simulink model "TEModel"  (Simulink 8.3)
settings: Solver=ode1  SolverMode=SingleTasking  StartTime=0.0  StopTime=72  FixedStep=Ts_base  MaxStep=Ts_base  MinStep=1e-6  RelTol=1e-6
PreLoadFcn:
  | initModel
StopFcn:
  | TEplot
undefined symbols (not defined in the file): Ts_base, Ts_save
libraries: VAlib x28, TElib x18
(part 8 of 9)

== system TEModel/TE Plant/xmeas atk block/xmeas11 attack controller/Attack Type Controller ==
  note: 1) Only subsystems can be added as variant choices at this level
      | 2) Blocks cannot be connected at this level as connectivity is
      | automatically determined at simulation, based on the active variant
  normal : Inport
  faked : Inport  Port=2
  interval forward controller : Subsystem  VariantControl=interval_forward_controller
      mask Display:
      | disp('IFC')
      | port_label('input', 1, 'normal in')
      | port_label('input', 2, 'faked in')
      | port_label('output', 1, 'out')
  normal forward controller : Subsystem  VariantControl=normal_forward_controller
      mask Display:
      | disp('NFC')
      | port_label('input', 1, 'normal in')
      | port_label('input', 2, 'faked in')
      | port_label('output', 1, 'out')
  periodical forward controller : Subsystem  VariantControl=periodical_forward_controller
      mask Display:
      | disp('PFC')
      | port_label('input', 1, 'normal in')
      | port_label('input', 2, 'faked in')
      | port_label('output', 1, 'out')
  step forward controller : Subsystem  VariantControl=step_forward_controller
      mask Display:
      | disp('SFC')
      | port_label('input', 1, 'normal in')
      | port_label('input', 2, 'faked in')
      | port_label('output', 1, 'out')
  output : Outport

== system TEModel/TE Plant/xmeas atk block/xmeas12 attack controller/Attack Type Controller ==
  note: 1) Only subsystems can be added as variant choices at this level
      | 2) Blocks cannot be connected at this level as connectivity is
      | automatically determined at simulation, based on the active variant
  normal : Inport
  faked : Inport  Port=2
  interval forward controller : Subsystem  VariantControl=interval_forward_controller
      mask Display:
      | disp('IFC')
      | port_label('input', 1, 'normal in')
      | port_label('input', 2, 'faked in')
      | port_label('output', 1, 'out')
  normal forward controller : Subsystem  VariantControl=normal_forward_controller
      mask Display:
      | disp('NFC')
      | port_label('input', 1, 'normal in')
      | port_label('input', 2, 'faked in')
      | port_label('output', 1, 'out')
  periodical forward controller : Subsystem  VariantControl=periodical_forward_controller
      mask Display:
      | disp('PFC')
      | port_label('input', 1, 'normal in')
      | port_label('input', 2, 'faked in')
      | port_label('output', 1, 'out')
  step forward controller : Subsystem  VariantControl=step_forward_controller
      mask Display:
      | disp('SFC')
      | port_label('input', 1, 'normal in')
      | port_label('input', 2, 'faked in')
      | port_label('output', 1, 'out')
  output : Outport

== system TEModel/TE Plant/xmeas atk block/xmeas14 attack controller/Attack Type Controller ==
  note: 1) Only subsystems can be added as variant choices at this level
      | 2) Blocks cannot be connected at this level as connectivity is
      | automatically determined at simulation, based on the active variant
  normal : Inport
  faked : Inport  Port=2
  interval forward controller : Subsystem  VariantControl=interval_forward_controller
      mask Display:
      | disp('IFC')
      | port_label('input', 1, 'normal in')
      | port_label('input', 2, 'faked in')
      | port_label('output', 1, 'out')
  normal forward controller : Subsystem  VariantControl=normal_forward_controller
      mask Display:
      | disp('NFC')
      | port_label('input', 1, 'normal in')
      | port_label('input', 2, 'faked in')
      | port_label('output', 1, 'out')
  periodical forward controller : Subsystem  VariantControl=periodical_forward_controller
      mask Display:
      | disp('PFC')
      | port_label('input', 1, 'normal in')
      | port_label('input', 2, 'faked in')
      | port_label('output', 1, 'out')
  step forward controller : Subsystem  VariantControl=step_forward_controller
      mask Display:
      | disp('SFC')
      | port_label('input', 1, 'normal in')
      | port_label('input', 2, 'faked in')
      | port_label('output', 1, 'out')
  output : Outport

== system TEModel/TE Plant/xmeas atk block/xmeas15 attack controller/Attack Type Controller ==
  note: 1) Only subsystems can be added as variant choices at this level
      | 2) Blocks cannot be connected at this level as connectivity is
      | automatically determined at simulation, based on the active variant
  normal : Inport
  faked : Inport  Port=2
  interval forward controller : Subsystem  VariantControl=interval_forward_controller
      mask Display:
      | disp('IFC')
      | port_label('input', 1, 'normal in')
      | port_label('input', 2, 'faked in')
      | port_label('output', 1, 'out')
  normal forward controller : Subsystem  VariantControl=normal_forward_controller
      mask Display:
      | disp('NFC')
      | port_label('input', 1, 'normal in')
      | port_label('input', 2, 'faked in')
      | port_label('output', 1, 'out')
  periodical forward controller : Subsystem  VariantControl=periodical_forward_controller
      mask Display:
      | disp('PFC')
      | port_label('input', 1, 'normal in')
      | port_label('input', 2, 'faked in')
      | port_label('output', 1, 'out')
  step forward controller : Subsystem  VariantControl=step_forward_controller
      mask Display:
      | disp('SFC')
      | port_label('input', 1, 'normal in')
      | port_label('input', 2, 'faked in')
      | port_label('output', 1, 'out')
  output : Outport

== system TEModel/TE Plant/xmeas atk block/xmeas17 attack controller/Attack Type Controller ==
  note: 1) Only subsystems can be added as variant choices at this level
      | 2) Blocks cannot be connected at this level as connectivity is
      | automatically determined at simulation, based on the active variant
  normal : Inport
  faked : Inport  Port=2
  interval forward controller : Subsystem  VariantControl=interval_forward_controller
      mask Display:
      | disp('IFC')
      | port_label('input', 1, 'normal in')
      | port_label('input', 2, 'faked in')
      | port_label('output', 1, 'out')
  normal forward controller : Subsystem  VariantControl=normal_forward_controller
      mask Display:
      | disp('NFC')
      | port_label('input', 1, 'normal in')
      | port_label('input', 2, 'faked in')
      | port_label('output', 1, 'out')
  periodical forward controller : Subsystem  VariantControl=periodical_forward_controller
      mask Display:
      | disp('PFC')
      | port_label('input', 1, 'normal in')
      | port_label('input', 2, 'faked in')
      | port_label('output', 1, 'out')
  step forward controller : Subsystem  VariantControl=step_forward_controller
      mask Display:
      | disp('SFC')
      | port_label('input', 1, 'normal in')
      | port_label('input', 2, 'faked in')
      | port_label('output', 1, 'out')
  output : Outport

== system TEModel/TE Plant/xmeas atk block/xmeas2 attack controller/Attack Type Controller ==
  note: 1) Only subsystems can be added as variant choices at this level
      | 2) Blocks cannot be connected at this level as connectivity is
      | automatically determined at simulation, based on the active variant
  normal : Inport
  faked : Inport  Port=2
  interval forward controller : Subsystem  VariantControl=interval_forward_controller
      mask Display:
      | disp('IFC')
      | port_label('input', 1, 'normal in')
      | port_label('input', 2, 'faked in')
      | port_label('output', 1, 'out')
  normal forward controller : Subsystem  VariantControl=normal_forward_controller
      mask Display:
      | disp('NFC')
      | port_label('input', 1, 'normal in')
      | port_label('input', 2, 'faked in')
      | port_label('output', 1, 'out')
  periodical forward controller : Subsystem  VariantControl=periodical_forward_controller
      mask Display:
      | disp('PFC')
      | port_label('input', 1, 'normal in')
      | port_label('input', 2, 'faked in')
      | port_label('output', 1, 'out')
  step forward controller : Subsystem  VariantControl=step_forward_controller
      mask Display:
      | disp('SFC')
      | port_label('input', 1, 'normal in')
      | port_label('input', 2, 'faked in')
      | port_label('output', 1, 'out')
  output : Outport

== system TEModel/TE Plant/xmeas atk block/xmeas3 attack controller/Attack Type Controller ==
  note: 1) Only subsystems can be added as variant choices at this level
      | 2) Blocks cannot be connected at this level as connectivity is
      | automatically determined at simulation, based on the active variant
  normal : Inport
  faked : Inport  Port=2
  interval forward controller : Subsystem  VariantControl=interval_forward_controller
      mask Display:
      | disp('IFC')
      | port_label('input', 1, 'normal in')
      | port_label('input', 2, 'faked in')
      | port_label('output', 1, 'out')
  normal forward controller : Subsystem  VariantControl=normal_forward_controller
      mask Display:
      | disp('NFC')
      | port_label('input', 1, 'normal in')
      | port_label('input', 2, 'faked in')
      | port_label('output', 1, 'out')
  periodical forward controller : Subsystem  VariantControl=periodical_forward_controller
      mask Display:
      | disp('PFC')
      | port_label('input', 1, 'normal in')
      | port_label('input', 2, 'faked in')
      | port_label('output', 1, 'out')
  step forward controller : Subsystem  VariantControl=step_forward_controller
      mask Display:
      | disp('SFC')
      | port_label('input', 1, 'normal in')
      | port_label('input', 2, 'faked in')
      | port_label('output', 1, 'out')
  output : Outport

== system TEModel/TE Plant/xmeas atk block/xmeas31 attack controller/Attack Type Controller ==
  note: 1) Only subsystems can be added as variant choices at this level
      | 2) Blocks cannot be connected at this level as connectivity is
      | automatically determined at simulation, based on the active variant
  normal : Inport
  faked : Inport  Port=2
  interval forward controller : Subsystem  VariantControl=interval_forward_controller
      mask Display:
      | disp('IFC')
      | port_label('input', 1, 'normal in')
      | port_label('input', 2, 'faked in')
      | port_label('output', 1, 'out')
  normal forward controller : Subsystem  VariantControl=normal_forward_controller
      mask Display:
      | disp('NFC')
      | port_label('input', 1, 'normal in')
      | port_label('input', 2, 'faked in')
      | port_label('output', 1, 'out')
  periodical forward controller : Subsystem  VariantControl=periodical_forward_controller
      mask Display:
      | disp('PFC')
      | port_label('input', 1, 'normal in')
      | port_label('input', 2, 'faked in')
      | port_label('output', 1, 'out')
  step forward controller : Subsystem  VariantControl=step_forward_controller
      mask Display:
      | disp('SFC')
      | port_label('input', 1, 'normal in')
      | port_label('input', 2, 'faked in')
      | port_label('output', 1, 'out')
  output : Outport

== system TEModel/TE Plant/xmeas atk block/xmeas4 attack controller/Attack Type Controller ==
  note: 1) Only subsystems can be added as variant choices at this level
      | 2) Blocks cannot be connected at this level as connectivity is
      | automatically determined at simulation, based on the active variant
  normal : Inport
  faked : Inport  Port=2
  interval forward controller : Subsystem  VariantControl=interval_forward_controller
      mask Display:
      | disp('IFC')
      | port_label('input', 1, 'normal in')
      | port_label('input', 2, 'faked in')
      | port_label('output', 1, 'out')
  normal forward controller : Subsystem  VariantControl=normal_forward_controller
      mask Display:
      | disp('NFC')
      | port_label('input', 1, 'normal in')
      | port_label('input', 2, 'faked in')
      | port_label('output', 1, 'out')
  periodical forward controller : Subsystem  VariantControl=periodical_forward_controller
      mask Display:
      | disp('PFC')
      | port_label('input', 1, 'normal in')
      | port_label('input', 2, 'faked in')
      | port_label('output', 1, 'out')
  step forward controller : Subsystem  VariantControl=step_forward_controller
      mask Display:
      | disp('SFC')
      | port_label('input', 1, 'normal in')
      | port_label('input', 2, 'faked in')
      | port_label('output', 1, 'out')
  output : Outport

== system TEModel/TE Plant/xmeas atk block/xmeas40 attack controller/Attack Type Controller ==
  note: 1) Only subsystems can be added as variant choices at this level
      | 2) Blocks cannot be connected at this level as connectivity is
      | automatically determined at simulation, based on the active variant
  normal : Inport
  faked : Inport  Port=2
  interval forward controller : Subsystem  VariantControl=interval_forward_controller
      mask Display:
      | disp('IFC')
      | port_label('input', 1, 'normal in')
      | port_label('input', 2, 'faked in')
      | port_label('output', 1, 'out')
  normal forward controller : Subsystem  VariantControl=normal_forward_controller
      mask Display:
      | disp('NFC')
      | port_label('input', 1, 'normal in')
      | port_label('input', 2, 'faked in')
      | port_label('output', 1, 'out')
  periodical forward controller : Subsystem  VariantControl=periodical_forward_controller
      mask Display:
      | disp('PFC')
      | port_label('input', 1, 'normal in')
      | port_label('input', 2, 'faked in')
      | port_label('output', 1, 'out')
  step forward controller : Subsystem  VariantControl=step_forward_controller
      mask Display:
      | disp('SFC')
      | port_label('input', 1, 'normal in')
      | port_label('input', 2, 'faked in')
      | port_label('output', 1, 'out')
  output : Outport

== system TEModel/TE Plant/xmeas atk block/xmeas5 attack controller/Attack Type Controller ==
  note: 1) Only subsystems can be added as variant choices at this level
      | 2) Blocks cannot be connected at this level as connectivity is
      | automatically determined at simulation, based on the active variant
  normal : Inport
  faked : Inport  Port=2
  interval forward controller : Subsystem  VariantControl=interval_forward_controller
      mask Display:
      | disp('IFC')
      | port_label('input', 1, 'normal in')
      | port_label('input', 2, 'faked in')
      | port_label('output', 1, 'out')
  normal forward controller : Subsystem  VariantControl=normal_forward_controller
      mask Display:
      | disp('NFC')
      | port_label('input', 1, 'normal in')
      | port_label('input', 2, 'faked in')
      | port_label('output', 1, 'out')
  periodical forward controller : Subsystem  VariantControl=periodical_forward_controller
      mask Display:
      | disp('PFC')
      | port_label('input', 1, 'normal in')
      | port_label('input', 2, 'faked in')
      | port_label('output', 1, 'out')
  step forward controller : Subsystem  VariantControl=step_forward_controller
      mask Display:
      | disp('SFC')
      | port_label('input', 1, 'normal in')
      | port_label('input', 2, 'faked in')
      | port_label('output', 1, 'out')
  output : Outport

== system TEModel/TE Plant/xmeas atk block/xmeas7 attack controller/Attack Type Controller ==
  note: 1) Only subsystems can be added as variant choices at this level
      | 2) Blocks cannot be connected at this level as connectivity is
      | automatically determined at simulation, based on the active variant
  normal : Inport
  faked : Inport  Port=2
  interval forward controller : Subsystem  VariantControl=interval_forward_controller
      mask Display:
      | disp('IFC')
      | port_label('input', 1, 'normal in')
      | port_label('input', 2, 'faked in')
      | port_label('output', 1, 'out')
  normal forward controller : Subsystem  VariantControl=normal_forward_controller
      mask Display:
      | disp('NFC')
      | port_label('input', 1, 'normal in')
      | port_label('input', 2, 'faked in')
      | port_label('output', 1, 'out')
  periodical forward controller : Subsystem  VariantControl=periodical_forward_controller
      mask Display:
      | disp('PFC')
      | port_label('input', 1, 'normal in')
      | port_label('input', 2, 'faked in')
      | port_label('output', 1, 'out')
  step forward controller : Subsystem  VariantControl=step_forward_controller
      mask Display:
      | disp('SFC')
      | port_label('input', 1, 'normal in')
      | port_label('input', 2, 'faked in')
      | port_label('output', 1, 'out')
  output : Outport

== system TEModel/TE Plant/xmeas atk block/xmeas8 attack controller/Attack Type Controller ==
  note: 1) Only subsystems can be added as variant choices at this level
      | 2) Blocks cannot be connected at this level as connectivity is
      | automatically determined at simulation, based on the active variant
  normal : Inport
  faked : Inport  Port=2
  interval forward controller : Subsystem  VariantControl=interval_forward_controller
      mask Display:
      | disp('IFC')
      | port_label('input', 1, 'normal in')
      | port_label('input', 2, 'faked in')
      | port_label('output', 1, 'out')
  normal forward controller : Subsystem  VariantControl=normal_forward_controller
      mask Display:
      | disp('NFC')
      | port_label('input', 1, 'normal in')
      | port_label('input', 2, 'faked in')
      | port_label('output', 1, 'out')
  periodical forward controller : Subsystem  VariantControl=periodical_forward_controller
      mask Display:
      | disp('PFC')
      | port_label('input', 1, 'normal in')
      | port_label('input', 2, 'faked in')
      | port_label('output', 1, 'out')
  step forward controller : Subsystem  VariantControl=step_forward_controller
      mask Display:
      | disp('SFC')
      | port_label('input', 1, 'normal in')
      | port_label('input', 2, 'faked in')
      | port_label('output', 1, 'out')
  output : Outport

== system TEModel/TE Plant/xmeas atk block/xmeas9 attack controller/Attack Type Controller ==
  note: 1) Only subsystems can be added as variant choices at this level
      | 2) Blocks cannot be connected at this level as connectivity is
      | automatically determined at simulation, based on the active variant
  normal : Inport
  faked : Inport  Port=2
  interval forward controller : Subsystem  VariantControl=interval_forward_controller
      mask Display:
      | disp('IFC')
      | port_label('input', 1, 'normal in')
      | port_label('input', 2, 'faked in')
      | port_label('output', 1, 'out')
  normal forward controller : Subsystem  VariantControl=normal_forward_controller
      mask Display:
      | disp('NFC')
      | port_label('input', 1, 'normal in')
      | port_label('input', 2, 'faked in')
      | port_label('output', 1, 'out')
  periodical forward controller : Subsystem  VariantControl=periodical_forward_controller
      mask Display:
      | disp('PFC')
      | port_label('input', 1, 'normal in')
      | port_label('input', 2, 'faked in')
      | port_label('output', 1, 'out')
  step forward controller : Subsystem  VariantControl=step_forward_controller
      mask Display:
      | disp('SFC')
      | port_label('input', 1, 'normal in')
      | port_label('input', 2, 'faked in')
      | port_label('output', 1, 'out')
  output : Outport

== system TEModel/TE Plant/xmv atk block/xmv1 attack controller/Attack Type Controller ==
  note: 1) Only subsystems can be added as variant choices at this level
      | 2) Blocks cannot be connected at this level as connectivity is
      | automatically determined at simulation, based on the active variant
  normal : Inport
  faked : Inport  Port=2
  interval forward controller : Subsystem  VariantControl=interval_forward_controller
      mask Display:
      | disp('IFC')
      | port_label('input', 1, 'normal in')
      | port_label('input', 2, 'faked in')
      | port_label('output', 1, 'out')
  normal forward controller : Subsystem  VariantControl=normal_forward_controller
      mask Display:
      | disp('NFC')
      | port_label('input', 1, 'normal in')
      | port_label('input', 2, 'faked in')
      | port_label('output', 1, 'out')
  periodical forward controller : Subsystem  VariantControl=periodical_forward_controller
      mask Display:
      | disp('PFC')
      | port_label('input', 1, 'normal in')
      | port_label('input', 2, 'faked in')
      | port_label('output', 1, 'out')
  step forward controller : Subsystem  VariantControl=step_forward_controller
      mask Display:
      | disp('SFC')
      | port_label('input', 1, 'normal in')
      | port_label('input', 2, 'faked in')
      | port_label('output', 1, 'out')
  output : Outport

== system TEModel/TE Plant/xmv atk block/xmv10 attack controller/Attack Type Controller ==
  note: 1) Only subsystems can be added as variant choices at this level
      | 2) Blocks cannot be connected at this level as connectivity is
      | automatically determined at simulation, based on the active variant
  normal : Inport
  faked : Inport  Port=2
  interval forward controller : Subsystem  VariantControl=interval_forward_controller
      mask Display:
      | disp('IFC')
      | port_label('input', 1, 'normal in')
      | port_label('input', 2, 'faked in')
      | port_label('output', 1, 'out')
  normal forward controller : Subsystem  VariantControl=normal_forward_controller
      mask Display:
      | disp('NFC')
      | port_label('input', 1, 'normal in')
      | port_label('input', 2, 'faked in')
      | port_label('output', 1, 'out')
  periodical forward controller : Subsystem  VariantControl=periodical_forward_controller
      mask Display:
      | disp('PFC')
      | port_label('input', 1, 'normal in')
      | port_label('input', 2, 'faked in')
      | port_label('output', 1, 'out')
  step forward controller : Subsystem  VariantControl=step_forward_controller
      mask Display:
      | disp('SFC')
      | port_label('input', 1, 'normal in')
      | port_label('input', 2, 'faked in')
      | port_label('output', 1, 'out')
  output : Outport

== system TEModel/TE Plant/xmv atk block/xmv11 attack controller/Attack Type Controller ==
  note: 1) Only subsystems can be added as variant choices at this level
      | 2) Blocks cannot be connected at this level as connectivity is
      | automatically determined at simulation, based on the active variant
  normal : Inport
  faked : Inport  Port=2
  interval forward controller : Subsystem  VariantControl=interval_forward_controller
      mask Display:
      | disp('IFC')
      | port_label('input', 1, 'normal in')
      | port_label('input', 2, 'faked in')
      | port_label('output', 1, 'out')
  normal forward controller : Subsystem  VariantControl=normal_forward_controller
      mask Display:
      | disp('NFC')
      | port_label('input', 1, 'normal in')
      | port_label('input', 2, 'faked in')
      | port_label('output', 1, 'out')
  periodical forward controller : Subsystem  VariantControl=periodical_forward_controller
      mask Display:
      | disp('PFC')
      | port_label('input', 1, 'normal in')
      | port_label('input', 2, 'faked in')
      | port_label('output', 1, 'out')
  step forward controller : Subsystem  VariantControl=step_forward_controller
      mask Display:
      | disp('SFC')
      | port_label('input', 1, 'normal in')
      | port_label('input', 2, 'faked in')
      | port_label('output', 1, 'out')
  output : Outport

== system TEModel/TE Plant/xmv atk block/xmv12 attack controller/Attack Type Controller ==
  note: 1) Only subsystems can be added as variant choices at this level
      | 2) Blocks cannot be connected at this level as connectivity is
      | automatically determined at simulation, based on the active variant
  normal : Inport
  faked : Inport  Port=2
  interval forward controller : Subsystem  VariantControl=interval_forward_controller
      mask Display:
      | disp('IFC')
      | port_label('input', 1, 'normal in')
      | port_label('input', 2, 'faked in')
      | port_label('output', 1, 'out')
  normal forward controller : Subsystem  VariantControl=normal_forward_controller
      mask Display:
      | disp('NFC')
      | port_label('input', 1, 'normal in')
      | port_label('input', 2, 'faked in')
      | port_label('output', 1, 'out')
  periodical forward controller : Subsystem  VariantControl=periodical_forward_controller
      mask Display:
      | disp('PFC')
      | port_label('input', 1, 'normal in')
      | port_label('input', 2, 'faked in')
      | port_label('output', 1, 'out')
  step forward controller : Subsystem  VariantControl=step_forward_controller
      mask Display:
      | disp('SFC')
      | port_label('input', 1, 'normal in')
      | port_label('input', 2, 'faked in')
      | port_label('output', 1, 'out')
  output : Outport

== system TEModel/TE Plant/xmv atk block/xmv2 attack controller/Attack Type Controller ==
  note: 1) Only subsystems can be added as variant choices at this level
      | 2) Blocks cannot be connected at this level as connectivity is
      | automatically determined at simulation, based on the active variant
  normal : Inport
  faked : Inport  Port=2
  interval forward controller : Subsystem  VariantControl=interval_forward_controller
      mask Display:
      | disp('IFC')
      | port_label('input', 1, 'normal in')
      | port_label('input', 2, 'faked in')
      | port_label('output', 1, 'out')
  normal forward controller : Subsystem  VariantControl=normal_forward_controller
      mask Display:
      | disp('NFC')
      | port_label('input', 1, 'normal in')
      | port_label('input', 2, 'faked in')
      | port_label('output', 1, 'out')
  periodical forward controller : Subsystem  VariantControl=periodical_forward_controller
      mask Display:
      | disp('PFC')
      | port_label('input', 1, 'normal in')
      | port_label('input', 2, 'faked in')
      | port_label('output', 1, 'out')
  step forward controller : Subsystem  VariantControl=step_forward_controller
      mask Display:
      | disp('SFC')
      | port_label('input', 1, 'normal in')
      | port_label('input', 2, 'faked in')
      | port_label('output', 1, 'out')
  output : Outport

== system TEModel/TE Plant/xmv atk block/xmv3 attack controller/Attack Type Controller ==
  note: 1) Only subsystems can be added as variant choices at this level
      | 2) Blocks cannot be connected at this level as connectivity is
      | automatically determined at simulation, based on the active variant
  normal : Inport
  faked : Inport  Port=2
  interval forward controller : Subsystem  VariantControl=interval_forward_controller
      mask Display:
      | disp('IFC')
      | port_label('input', 1, 'normal in')
      | port_label('input', 2, 'faked in')
      | port_label('output', 1, 'out')
  normal forward controller : Subsystem  VariantControl=normal_forward_controller
      mask Display:
      | disp('NFC')
      | port_label('input', 1, 'normal in')
      | port_label('input', 2, 'faked in')
      | port_label('output', 1, 'out')
  periodical forward controller : Subsystem  VariantControl=periodical_forward_controller
      mask Display:
      | disp('PFC')
      | port_label('input', 1, 'normal in')
      | port_label('input', 2, 'faked in')
      | port_label('output', 1, 'out')
  step forward controller : Subsystem  VariantControl=step_forward_controller
      mask Display:
      | disp('SFC')
      | port_label('input', 1, 'normal in')
      | port_label('input', 2, 'faked in')
      | port_label('output', 1, 'out')
  output : Outport

== system TEModel/TE Plant/xmv atk block/xmv4 attack controller/Attack Type Controller ==
  note: 1) Only subsystems can be added as variant choices at this level
      | 2) Blocks cannot be connected at this level as connectivity is
      | automatically determined at simulation, based on the active variant
  normal : Inport
  faked : Inport  Port=2
  interval forward controller : Subsystem  VariantControl=interval_forward_controller
      mask Display:
      | disp('IFC')
      | port_label('input', 1, 'normal in')
      | port_label('input', 2, 'faked in')
      | port_label('output', 1, 'out')
  normal forward controller : Subsystem  VariantControl=normal_forward_controller
      mask Display:
      | disp('NFC')
      | port_label('input', 1, 'normal in')
      | port_label('input', 2, 'faked in')
      | port_label('output', 1, 'out')
  periodical forward controller : Subsystem  VariantControl=periodical_forward_controller
      mask Display:
      | disp('PFC')
      | port_label('input', 1, 'normal in')
      | port_label('input', 2, 'faked in')
      | port_label('output', 1, 'out')
  step forward controller : Subsystem  VariantControl=step_forward_controller
      mask Display:
      | disp('SFC')
      | port_label('input', 1, 'normal in')
      | port_label('input', 2, 'faked in')
      | port_label('output', 1, 'out')
  output : Outport

== system TEModel/TE Plant/xmv atk block/xmv5 attack controller/Attack Type Controller ==
  note: 1) Only subsystems can be added as variant choices at this level
      | 2) Blocks cannot be connected at this level as connectivity is
      | automatically determined at simulation, based on the active variant
  normal : Inport
  faked : Inport  Port=2
  interval forward controller : Subsystem  VariantControl=interval_forward_controller
      mask Display:
      | disp('IFC')
      | port_label('input', 1, 'normal in')
      | port_label('input', 2, 'faked in')
      | port_label('output', 1, 'out')
  normal forward controller : Subsystem  VariantControl=normal_forward_controller
      mask Display:
      | disp('NFC')
      | port_label('input', 1, 'normal in')
      | port_label('input', 2, 'faked in')
      | port_label('output', 1, 'out')
  periodical forward controller : Subsystem  VariantControl=periodical_forward_controller
      mask Display:
      | disp('PFC')
      | port_label('input', 1, 'normal in')
      | port_label('input', 2, 'faked in')
      | port_label('output', 1, 'out')
  step forward controller : Subsystem  VariantControl=step_forward_controller
      mask Display:
      | disp('SFC')
      | port_label('input', 1, 'normal in')
      | port_label('input', 2, 'faked in')
      | port_label('output', 1, 'out')
  output : Outport

== system TEModel/TE Plant/xmv atk block/xmv6 attack controller/Attack Type Controller ==
  note: 1) Only subsystems can be added as variant choices at this level
      | 2) Blocks cannot be connected at this level as connectivity is
      | automatically determined at simulation, based on the active variant
  normal : Inport
  faked : Inport  Port=2
  interval forward controller : Subsystem  VariantControl=interval_forward_controller
      mask Display:
      | disp('IFC')
      | port_label('input', 1, 'normal in')
      | port_label('input', 2, 'faked in')
      | port_label('output', 1, 'out')
  normal forward controller : Subsystem  VariantControl=normal_forward_controller
      mask Display:
      | disp('NFC')
      | port_label('input', 1, 'normal in')
      | port_label('input', 2, 'faked in')
      | port_label('output', 1, 'out')
  periodical forward controller : Subsystem  VariantControl=periodical_forward_controller
      mask Display:
      | disp('PFC')
      | port_label('input', 1, 'normal in')
      | port_label('input', 2, 'faked in')
      | port_label('output', 1, 'out')
  step forward controller : Subsystem  VariantControl=step_forward_controller
      mask Display:
      | disp('SFC')
      | port_label('input', 1, 'normal in')
      | port_label('input', 2, 'faked in')
      | port_label('output', 1, 'out')
  output : Outport

== system TEModel/TE Plant/xmv atk block/xmv7 attack controller/Attack Type Controller ==
  note: 1) Only subsystems can be added as variant choices at this level
      | 2) Blocks cannot be connected at this level as connectivity is
      | automatically determined at simulation, based on the active variant
  normal : Inport
  faked : Inport  Port=2
  interval forward controller : Subsystem  VariantControl=interval_forward_controller
      mask Display:
      | disp('IFC')
      | port_label('input', 1, 'normal in')
      | port_label('input', 2, 'faked in')
      | port_label('output', 1, 'out')
  normal forward controller : Subsystem  VariantControl=normal_forward_controller
      mask Display:
      | disp('NFC')
      | port_label('input', 1, 'normal in')
      | port_label('input', 2, 'faked in')
      | port_label('output', 1, 'out')
  periodical forward controller : Subsystem  VariantControl=periodical_forward_controller
      mask Display:
      | disp('PFC')
      | port_label('input', 1, 'normal in')
      | port_label('input', 2, 'faked in')
      | port_label('output', 1, 'out')
  step forward controller : Subsystem  VariantControl=step_forward_controller
      mask Display:
      | disp('SFC')
      | port_label('input', 1, 'normal in')
      | port_label('input', 2, 'faked in')
      | port_label('output', 1, 'out')
  output : Outport

== system TEModel/TE Plant/xmv atk block/xmv8 attack controller/Attack Type Controller ==
  note: 1) Only subsystems can be added as variant choices at this level
      | 2) Blocks cannot be connected at this level as connectivity is
      | automatically determined at simulation, based on the active variant
  normal : Inport
  faked : Inport  Port=2
  interval forward controller : Subsystem  VariantControl=interval_forward_controller
      mask Display:
      | disp('IFC')
      | port_label('input', 1, 'normal in')
      | port_label('input', 2, 'faked in')
      | port_label('output', 1, 'out')
  normal forward controller : Subsystem  VariantControl=normal_forward_controller
      mask Display:
      | disp('NFC')
      | port_label('input', 1, 'normal in')
      | port_label('input', 2, 'faked in')
      | port_label('output', 1, 'out')
  periodical forward controller : Subsystem  VariantControl=periodical_forward_controller
      mask Display:
      | disp('PFC')
      | port_label('input', 1, 'normal in')
      | port_label('input', 2, 'faked in')
      | port_label('output', 1, 'out')
  step forward controller : Subsystem  VariantControl=step_forward_controller
      mask Display:
      | disp('SFC')
      | port_label('input', 1, 'normal in')
      | port_label('input', 2, 'faked in')
      | port_label('output', 1, 'out')
  output : Outport

== system TEModel/TE Plant/xmv atk block/xmv9 attack controller/Attack Type Controller ==
  note: 1) Only subsystems can be added as variant choices at this level
      | 2) Blocks cannot be connected at this level as connectivity is
      | automatically determined at simulation, based on the active variant
  normal : Inport
  faked : Inport  Port=2
  interval forward controller : Subsystem  VariantControl=interval_forward_controller
      mask Display:
      | disp('IFC')
      | port_label('input', 1, 'normal in')
      | port_label('input', 2, 'faked in')
      | port_label('output', 1, 'out')
  normal forward controller : Subsystem  VariantControl=normal_forward_controller
      mask Display:
      | disp('NFC')
      | port_label('input', 1, 'normal in')
      | port_label('input', 2, 'faked in')
      | port_label('output', 1, 'out')
  periodical forward controller : Subsystem  VariantControl=periodical_forward_controller
      mask Display:
      | disp('PFC')
      | port_label('input', 1, 'normal in')
      | port_label('input', 2, 'faked in')
      | port_label('output', 1, 'out')
  step forward controller : Subsystem  VariantControl=step_forward_controller
      mask Display:
      | disp('SFC')
      | port_label('input', 1, 'normal in')
      | port_label('input', 2, 'faked in')
      | port_label('output', 1, 'out')
  output : Outport

== system TEModel/TE Plant/xmeas atk block/xmeas1 attack controller/Attack Type Controller/interval forward controller ==
  normal : Inport
  faked : Inport  Port=2
  Impuls : VAlib/Impuls  amplitude=1  duration=duration  delay=start
  Switch : Switch  Criteria=u2 > Threshold
  output : Outport
  wires:
  faked/1 -> Switch/1
  normal/1 -> Switch/3
  Impuls/1 -> Switch/2
  Switch/1 -> output/1

== system TEModel/TE Plant/xmeas atk block/xmeas1 attack controller/Attack Type Controller/normal forward controller ==
  normal : Inport
  faked : Inport  Port=2
  Terminator : Terminator
  output : Outport
  wires:
  normal/1 -> output/1
  faked/1 -> Terminator/1

== system TEModel/TE Plant/xmeas atk block/xmeas1 attack controller/Attack Type Controller/periodical forward controller ==
  normal : Inport
  faked : Inport  Port=2
  Pulse Generator : DiscretePulseGenerator  PulseType=Time based  Period=duration + start  PulseWidth=100*duration/(duration + start)  PhaseDelay=start
  Switch : Switch  Criteria=u2 > Threshold
  output : Outport
  wires:
  faked/1 -> Switch/1
  normal/1 -> Switch/3
  Pulse Generator/1 -> Switch/2
  Switch/1 -> output/1

== system TEModel/TE Plant/xmeas atk block/xmeas1 attack controller/Attack Type Controller/step forward controller ==
  normal : Inport
  faked : Inport  Port=2
  Step : Step  Time=start  SampleTime=0
  Switch : Switch  Criteria=u2 > Threshold
  output : Outport
  wires:
  faked/1 -> Switch/1
  normal/1 -> Switch/3
  Step/1 -> Switch/2
  Switch/1 -> output/1

== system TEModel/TE Plant/xmeas atk block/xmeas10 attack controller/Attack Type Controller/interval forward controller ==
  normal : Inport
  faked : Inport  Port=2
  Impuls : VAlib/Impuls  amplitude=1  duration=duration  delay=start
  Switch : Switch  Criteria=u2 > Threshold
  output : Outport
  wires:
  faked/1 -> Switch/1
  normal/1 -> Switch/3
  Impuls/1 -> Switch/2
  Switch/1 -> output/1

== system TEModel/TE Plant/xmeas atk block/xmeas10 attack controller/Attack Type Controller/normal forward controller ==
  normal : Inport
  faked : Inport  Port=2
  Terminator : Terminator
  output : Outport
  wires:
  normal/1 -> output/1
  faked/1 -> Terminator/1

== system TEModel/TE Plant/xmeas atk block/xmeas10 attack controller/Attack Type Controller/periodical forward controller ==
  normal : Inport
  faked : Inport  Port=2
  Pulse Generator : DiscretePulseGenerator  PulseType=Time based  Period=duration + start  PulseWidth=100*duration/(duration + start)  PhaseDelay=start
  Switch : Switch  Criteria=u2 > Threshold
  output : Outport
  wires:
  faked/1 -> Switch/1
  normal/1 -> Switch/3
  Pulse Generator/1 -> Switch/2
  Switch/1 -> output/1

== system TEModel/TE Plant/xmeas atk block/xmeas10 attack controller/Attack Type Controller/step forward controller ==
  normal : Inport
  faked : Inport  Port=2
  Step : Step  Time=start  SampleTime=0
  Switch : Switch  Criteria=u2 > Threshold
  output : Outport
  wires:
  faked/1 -> Switch/1
  normal/1 -> Switch/3
  Step/1 -> Switch/2
  Switch/1 -> output/1

== system TEModel/TE Plant/xmeas atk block/xmeas11 attack controller/Attack Type Controller/interval forward controller ==
  normal : Inport
  faked : Inport  Port=2
  Impuls : VAlib/Impuls  amplitude=1  duration=duration  delay=start
  Switch : Switch  Criteria=u2 > Threshold
  output : Outport
  wires:
  faked/1 -> Switch/1
  normal/1 -> Switch/3
  Impuls/1 -> Switch/2
  Switch/1 -> output/1

== system TEModel/TE Plant/xmeas atk block/xmeas11 attack controller/Attack Type Controller/normal forward controller ==
  normal : Inport
  faked : Inport  Port=2
  Terminator : Terminator
  output : Outport
  wires:
  normal/1 -> output/1
  faked/1 -> Terminator/1

== system TEModel/TE Plant/xmeas atk block/xmeas11 attack controller/Attack Type Controller/periodical forward controller ==
  normal : Inport
  faked : Inport  Port=2
  Pulse Generator : DiscretePulseGenerator  PulseType=Time based  Period=duration + start  PulseWidth=100*duration/(duration + start)  PhaseDelay=start
  Switch : Switch  Criteria=u2 > Threshold
  output : Outport
  wires:
  faked/1 -> Switch/1
  normal/1 -> Switch/3
  Pulse Generator/1 -> Switch/2
  Switch/1 -> output/1

== system TEModel/TE Plant/xmeas atk block/xmeas11 attack controller/Attack Type Controller/step forward controller ==
  normal : Inport
  faked : Inport  Port=2
  Step : Step  Time=start  SampleTime=0
  Switch : Switch  Criteria=u2 > Threshold
  output : Outport
  wires:
  faked/1 -> Switch/1
  normal/1 -> Switch/3
  Step/1 -> Switch/2
  Switch/1 -> output/1

== system TEModel/TE Plant/xmeas atk block/xmeas12 attack controller/Attack Type Controller/interval forward controller ==
  normal : Inport
  faked : Inport  Port=2
  Impuls : VAlib/Impuls  amplitude=1  duration=duration  delay=start
  Switch : Switch  Criteria=u2 > Threshold
  output : Outport
  wires:
  faked/1 -> Switch/1
  normal/1 -> Switch/3
  Impuls/1 -> Switch/2
  Switch/1 -> output/1

== system TEModel/TE Plant/xmeas atk block/xmeas12 attack controller/Attack Type Controller/normal forward controller ==
  normal : Inport
  faked : Inport  Port=2
  Terminator : Terminator
  output : Outport
  wires:
  normal/1 -> output/1
  faked/1 -> Terminator/1

== system TEModel/TE Plant/xmeas atk block/xmeas12 attack controller/Attack Type Controller/periodical forward controller ==
  normal : Inport
  faked : Inport  Port=2
  Pulse Generator : DiscretePulseGenerator  PulseType=Time based  Period=duration + start  PulseWidth=100*duration/(duration + start)  PhaseDelay=start
  Switch : Switch  Criteria=u2 > Threshold
  output : Outport
  wires:
  faked/1 -> Switch/1
  normal/1 -> Switch/3
  Pulse Generator/1 -> Switch/2
  Switch/1 -> output/1

== system TEModel/TE Plant/xmeas atk block/xmeas12 attack controller/Attack Type Controller/step forward controller ==
  normal : Inport
  faked : Inport  Port=2
  Step : Step  Time=start  SampleTime=0
  Switch : Switch  Criteria=u2 > Threshold
  output : Outport
  wires:
  faked/1 -> Switch/1
  normal/1 -> Switch/3
  Step/1 -> Switch/2
  Switch/1 -> output/1

== system TEModel/TE Plant/xmeas atk block/xmeas14 attack controller/Attack Type Controller/interval forward controller ==
  normal : Inport
  faked : Inport  Port=2
  Impuls : VAlib/Impuls  amplitude=1  duration=duration  delay=start
  Switch : Switch  Criteria=u2 > Threshold
  output : Outport
  wires:
  faked/1 -> Switch/1
  normal/1 -> Switch/3
  Impuls/1 -> Switch/2
  Switch/1 -> output/1

== system TEModel/TE Plant/xmeas atk block/xmeas14 attack controller/Attack Type Controller/normal forward controller ==
  normal : Inport
  faked : Inport  Port=2
  Terminator : Terminator
  output : Outport
  wires:
  normal/1 -> output/1
  faked/1 -> Terminator/1

== system TEModel/TE Plant/xmeas atk block/xmeas14 attack controller/Attack Type Controller/periodical forward controller ==
  normal : Inport
  faked : Inport  Port=2
  Pulse Generator : DiscretePulseGenerator  PulseType=Time based  Period=duration + start  PulseWidth=100*duration/(duration + start)  PhaseDelay=start
  Switch : Switch  Criteria=u2 > Threshold
  output : Outport
  wires:
  faked/1 -> Switch/1
  normal/1 -> Switch/3
  Pulse Generator/1 -> Switch/2
  Switch/1 -> output/1

== system TEModel/TE Plant/xmeas atk block/xmeas14 attack controller/Attack Type Controller/step forward controller ==
  normal : Inport
  faked : Inport  Port=2
  Step : Step  Time=start  SampleTime=0
  Switch : Switch  Criteria=u2 > Threshold
  output : Outport
  wires:
  faked/1 -> Switch/1
  normal/1 -> Switch/3
  Step/1 -> Switch/2
  Switch/1 -> output/1

== system TEModel/TE Plant/xmeas atk block/xmeas15 attack controller/Attack Type Controller/interval forward controller ==
  normal : Inport
  faked : Inport  Port=2
  Impuls : VAlib/Impuls  amplitude=1  duration=duration  delay=start
  Switch : Switch  Criteria=u2 > Threshold
  output : Outport
  wires:
  faked/1 -> Switch/1
  normal/1 -> Switch/3
  Impuls/1 -> Switch/2
  Switch/1 -> output/1

== system TEModel/TE Plant/xmeas atk block/xmeas15 attack controller/Attack Type Controller/normal forward controller ==
  normal : Inport
  faked : Inport  Port=2
  Terminator : Terminator
  output : Outport
  wires:
  normal/1 -> output/1
  faked/1 -> Terminator/1

== system TEModel/TE Plant/xmeas atk block/xmeas15 attack controller/Attack Type Controller/periodical forward controller ==
  normal : Inport
  faked : Inport  Port=2
  Pulse Generator : DiscretePulseGenerator  PulseType=Time based  Period=duration + start  PulseWidth=100*duration/(duration + start)  PhaseDelay=start
  Switch : Switch  Criteria=u2 > Threshold
  output : Outport
  wires:
  faked/1 -> Switch/1
  normal/1 -> Switch/3
  Pulse Generator/1 -> Switch/2
  Switch/1 -> output/1

== system TEModel/TE Plant/xmeas atk block/xmeas15 attack controller/Attack Type Controller/step forward controller ==
  normal : Inport
  faked : Inport  Port=2
  Step : Step  Time=start  SampleTime=0
  Switch : Switch  Criteria=u2 > Threshold
  output : Outport
  wires:
  faked/1 -> Switch/1
  normal/1 -> Switch/3
  Step/1 -> Switch/2
  Switch/1 -> output/1

== system TEModel/TE Plant/xmeas atk block/xmeas17 attack controller/Attack Type Controller/interval forward controller ==
  normal : Inport
  faked : Inport  Port=2
  Impuls : VAlib/Impuls  amplitude=1  duration=duration  delay=start
  Switch : Switch  Criteria=u2 > Threshold
  output : Outport
  wires:
  faked/1 -> Switch/1
  normal/1 -> Switch/3
  Impuls/1 -> Switch/2
  Switch/1 -> output/1

== system TEModel/TE Plant/xmeas atk block/xmeas17 attack controller/Attack Type Controller/normal forward controller ==
  normal : Inport
  faked : Inport  Port=2
  Terminator : Terminator
  output : Outport
  wires:
  normal/1 -> output/1
  faked/1 -> Terminator/1

== system TEModel/TE Plant/xmeas atk block/xmeas17 attack controller/Attack Type Controller/periodical forward controller ==
  normal : Inport
  faked : Inport  Port=2
  Pulse Generator : DiscretePulseGenerator  PulseType=Time based  Period=duration + start  PulseWidth=100*duration/(duration + start)  PhaseDelay=start
  Switch : Switch  Criteria=u2 > Threshold
  output : Outport
  wires:
  faked/1 -> Switch/1
  normal/1 -> Switch/3
  Pulse Generator/1 -> Switch/2
  Switch/1 -> output/1

== system TEModel/TE Plant/xmeas atk block/xmeas17 attack controller/Attack Type Controller/step forward controller ==
  normal : Inport
  faked : Inport  Port=2
  Step : Step  Time=start  SampleTime=0
  Switch : Switch  Criteria=u2 > Threshold
  output : Outport
  wires:
  faked/1 -> Switch/1
  normal/1 -> Switch/3
  Step/1 -> Switch/2
  Switch/1 -> output/1

== system TEModel/TE Plant/xmeas atk block/xmeas2 attack controller/Attack Type Controller/interval forward controller ==
  normal : Inport
  faked : Inport  Port=2
  Impuls : VAlib/Impuls  amplitude=1  duration=duration  delay=start
  Switch : Switch  Criteria=u2 > Threshold
  output : Outport
  wires:
  faked/1 -> Switch/1
  normal/1 -> Switch/3
  Impuls/1 -> Switch/2
  Switch/1 -> output/1

== system TEModel/TE Plant/xmeas atk block/xmeas2 attack controller/Attack Type Controller/normal forward controller ==
  normal : Inport
  faked : Inport  Port=2
  Terminator : Terminator
  output : Outport
  wires:
  normal/1 -> output/1
  faked/1 -> Terminator/1

== system TEModel/TE Plant/xmeas atk block/xmeas2 attack controller/Attack Type Controller/periodical forward controller ==
  normal : Inport
  faked : Inport  Port=2
  Pulse Generator : DiscretePulseGenerator  PulseType=Time based  Period=duration + start  PulseWidth=100*duration/(duration + start)  PhaseDelay=start
  Switch : Switch  Criteria=u2 > Threshold
  output : Outport
  wires:
  faked/1 -> Switch/1
  normal/1 -> Switch/3
  Pulse Generator/1 -> Switch/2
  Switch/1 -> output/1

== system TEModel/TE Plant/xmeas atk block/xmeas2 attack controller/Attack Type Controller/step forward controller ==
  normal : Inport
  faked : Inport  Port=2
  Step : Step  Time=start  SampleTime=0
  Switch : Switch  Criteria=u2 > Threshold
  output : Outport
  wires:
  faked/1 -> Switch/1
  normal/1 -> Switch/3
  Step/1 -> Switch/2
  Switch/1 -> output/1

== system TEModel/TE Plant/xmeas atk block/xmeas3 attack controller/Attack Type Controller/interval forward controller ==
  normal : Inport
  faked : Inport  Port=2
  Impuls : VAlib/Impuls  amplitude=1  duration=duration  delay=start
  Switch : Switch  Criteria=u2 > Threshold
  output : Outport
  wires:
  faked/1 -> Switch/1
  normal/1 -> Switch/3
  Impuls/1 -> Switch/2
  Switch/1 -> output/1

== system TEModel/TE Plant/xmeas atk block/xmeas3 attack controller/Attack Type Controller/normal forward controller ==
  normal : Inport
  faked : Inport  Port=2
  Terminator : Terminator
  output : Outport
  wires:
  normal/1 -> output/1
  faked/1 -> Terminator/1

== system TEModel/TE Plant/xmeas atk block/xmeas3 attack controller/Attack Type Controller/periodical forward controller ==
  normal : Inport
  faked : Inport  Port=2
  Pulse Generator : DiscretePulseGenerator  PulseType=Time based  Period=duration + start  PulseWidth=100*duration/(duration + start)  PhaseDelay=start
  Switch : Switch  Criteria=u2 > Threshold
  output : Outport
  wires:
  faked/1 -> Switch/1
  normal/1 -> Switch/3
  Pulse Generator/1 -> Switch/2
  Switch/1 -> output/1

== system TEModel/TE Plant/xmeas atk block/xmeas3 attack controller/Attack Type Controller/step forward controller ==
  normal : Inport
  faked : Inport  Port=2
  Step : Step  Time=start  SampleTime=0
  Switch : Switch  Criteria=u2 > Threshold
  output : Outport
  wires:
  faked/1 -> Switch/1
  normal/1 -> Switch/3
  Step/1 -> Switch/2
  Switch/1 -> output/1

== system TEModel/TE Plant/xmeas atk block/xmeas31 attack controller/Attack Type Controller/interval forward controller ==
  normal : Inport
  faked : Inport  Port=2
  Impuls : VAlib/Impuls  amplitude=1  duration=duration  delay=start
  Switch : Switch  Criteria=u2 > Threshold
  output : Outport
  wires:
  faked/1 -> Switch/1
  normal/1 -> Switch/3
  Impuls/1 -> Switch/2
  Switch/1 -> output/1
